simulink model "k1vispr2"  (Simulink 8.8)
settings: Solver=ode45  StartTime=0.0  StopTime=10.0  RelTol=1e-3  EnableMultiTasking=on
libraries: cdsEpicsBinIn x38, cdsEpicsOut x14, cdsBit2Word x14, cdsIPCx x12, cdsCDI64 x7, cdsCDO64 x7, cdsWord2Bit x6, dac x2, cdsAdcx0 x1, cdsCDO32 x1, TYPEBP_MASTER x1, BO_TYPEBP_MASTER x1
(part 2 of 3)

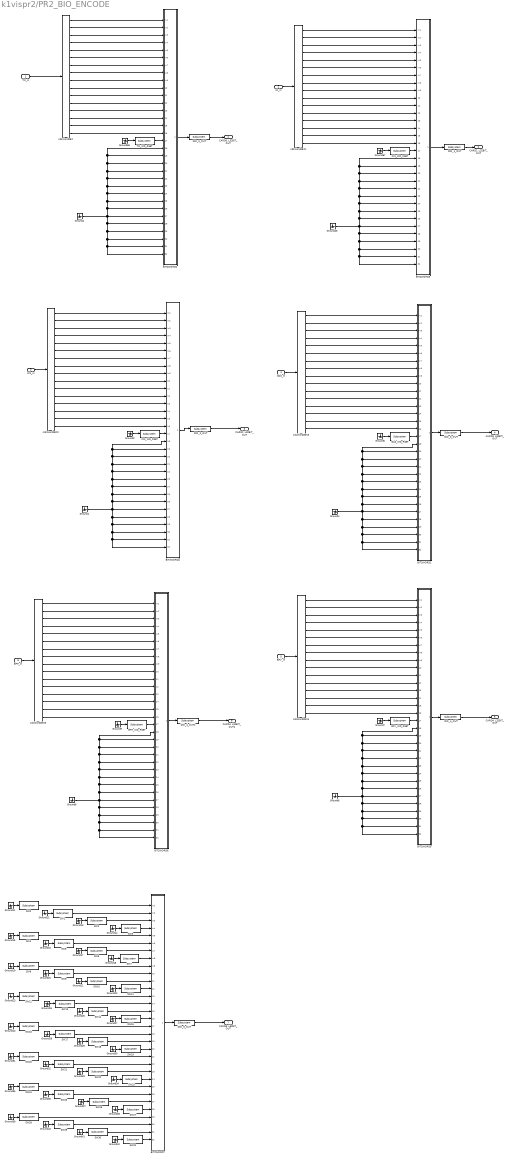
== system k1vispr2/PR2_BIO_ENCODE ==
  TM_In : Inport
  IM_In : Inport  Port=2
  IM1_In : Inport  Port=3
  GAS_In : Inport  Port=4
  BFV_In : Inport  Port=5
  BFH_In : Inport  Port=6
  BFH_WD_RSET : cdsEpicsBinIn/Subsystem  Tag=cdsEpicsBinIn  Description=|
      | Purpose:                                                                            
      | Create an EPICS binary (0 or 1) input channel to the FE realtime controls.          
      |                                                                                     
      | Operation:                                                                          
      | Outputs value from an EPICS ai record. Value is binary input (bi Epics record type).
      |                                                                                     
      | Usage:                                                                              
      | Name the part with the desired EPICS channel name.
      settings: AttributesFormatString=%<Tag>
  BFV_WD_RSET : cdsEpicsBinIn/Subsystem  Tag=cdsEpicsBinIn  Description=|
      | Purpose:                                                                            
      | Create an EPICS binary (0 or 1) input channel to the FE realtime controls.          
      |                                                                                     
      | Operation:                                                                          
      | Outputs value from an EPICS ai record. Value is binary input (bi Epics record type).
      |                                                                                     
      | Usage:                                                                              
      | Name the part with the desired EPICS channel name.
      settings: AttributesFormatString=%<Tag>
  BIT2WORD1 : Subsystem
  BIT2WORD2 : Subsystem
  BIT2WORD3 : Subsystem
  BIT2WORD4 : Subsystem
  BIT2WORD5 : Subsystem
  BIT2WORD6 : Subsystem
  BIT2WORD7 : Subsystem
  DIO_0_OUT : cdsEpicsOut/Subsystem  Tag=cdsEpicsOutput  Description=|
      | Purpose:                                          
      | Output a FE signal to an EPICS channel.           
      |                                                   
      | Operation:                                        
      | Takes input value and passes it to EPICS record.  
      |                                                   
      | Usage:                                            
      | Name the part with the desired EPICS rrecord name.
      settings: AttributesFormatString=%<Tag>
  DIO_1_OUT : cdsEpicsOut/Subsystem  Tag=cdsEpicsOutput  Description=|
      | Purpose:                                          
      | Output a FE signal to an EPICS channel.           
      |                                                   
      | Operation:                                        
      | Takes input value and passes it to EPICS record.  
      |                                                   
      | Usage:                                            
      | Name the part with the desired EPICS rrecord name.
      settings: AttributesFormatString=%<Tag>
  DIO_2_OUT : cdsEpicsOut/Subsystem  Tag=cdsEpicsOutput  Description=|
      | Purpose:                                          
      | Output a FE signal to an EPICS channel.           
      |                                                   
      | Operation:                                        
      | Takes input value and passes it to EPICS record.  
      |                                                   
      | Usage:                                            
      | Name the part with the desired EPICS rrecord name.
      settings: AttributesFormatString=%<Tag>
  DIO_3_OUT : cdsEpicsOut/Subsystem  Tag=cdsEpicsOutput  Description=|
      | Purpose:                                          
      | Output a FE signal to an EPICS channel.           
      |                                                   
      | Operation:                                        
      | Takes input value and passes it to EPICS record.  
      |                                                   
      | Usage:                                            
      | Name the part with the desired EPICS rrecord name.
      settings: AttributesFormatString=%<Tag>
  DIO_4_OUT : cdsEpicsOut/Subsystem  Tag=cdsEpicsOutput  Description=|
      | Purpose:                                          
      | Output a FE signal to an EPICS channel.           
      |                                                   
      | Operation:                                        
      | Takes input value and passes it to EPICS record.  
      |                                                   
      | Usage:                                            
      | Name the part with the desired EPICS rrecord name.
      settings: AttributesFormatString=%<Tag>
  DIO_4_OUT1 : cdsEpicsOut/Subsystem  Tag=cdsEpicsOutput  Description=|
      | Purpose:                                          
      | Output a FE signal to an EPICS channel.           
      |                                                   
      | Operation:                                        
      | Takes input value and passes it to EPICS record.  
      |                                                   
      | Usage:                                            
      | Name the part with the desired EPICS rrecord name.
      settings: AttributesFormatString=%<Tag>
  DIO_6_OUT : cdsEpicsOut/Subsystem  Tag=cdsEpicsOutput  Description=|
      | Purpose:                                          
      | Output a FE signal to an EPICS channel.           
      |                                                   
      | Operation:                                        
      | Takes input value and passes it to EPICS record.  
      |                                                   
      | Usage:                                            
      | Name the part with the desired EPICS rrecord name.
      settings: AttributesFormatString=%<Tag>
  GAS_WD_RSET : cdsEpicsBinIn/Subsystem  Tag=cdsEpicsBinIn  Description=|
      | Purpose:                                                                            
      | Create an EPICS binary (0 or 1) input channel to the FE realtime controls.          
      |                                                                                     
      | Operation:                                                                          
      | Outputs value from an EPICS ai record. Value is binary input (bi Epics record type).
      |                                                                                     
      | Usage:                                                                              
      | Name the part with the desired EPICS channel name.
      settings: AttributesFormatString=%<Tag>
  Ground{1..42,66..67} (44 alike) : Ground
  IM1_WD_RSET : cdsEpicsBinIn/Subsystem  Tag=cdsEpicsBinIn  Description=|
      | Purpose:                                                                            
      | Create an EPICS binary (0 or 1) input channel to the FE realtime controls.          
      |                                                                                     
      | Operation:                                                                          
      | Outputs value from an EPICS ai record. Value is binary input (bi Epics record type).
      |                                                                                     
      | Usage:                                                                              
      | Name the part with the desired EPICS channel name.
      settings: AttributesFormatString=%<Tag>
  IM2_WD_RSET : cdsEpicsBinIn/Subsystem  Tag=cdsEpicsBinIn  Description=|
      | Purpose:                                                                            
      | Create an EPICS binary (0 or 1) input channel to the FE realtime controls.          
      |                                                                                     
      | Operation:                                                                          
      | Outputs value from an EPICS ai record. Value is binary input (bi Epics record type).
      |                                                                                     
      | Usage:                                                                              
      | Name the part with the desired EPICS channel name.
      settings: AttributesFormatString=%<Tag>
  SW0 : cdsEpicsBinIn/Subsystem  Tag=cdsEpicsBinIn  Description=|
      | Purpose:                                                                            
      | Create an EPICS binary (0 or 1) input channel to the FE realtime controls.          
      |                                                                                     
      | Operation:                                                                          
      | Outputs value from an EPICS ai record. Value is binary input (bi Epics record type).
      |                                                                                     
      | Usage:                                                                              
      | Name the part with the desired EPICS channel name.
      settings: AttributesFormatString=%<Tag>
  SW1 : cdsEpicsBinIn/Subsystem  Tag=cdsEpicsBinIn  Description=|
      | Purpose:                                                                            
      | Create an EPICS binary (0 or 1) input channel to the FE realtime controls.          
      |                                                                                     
      | Operation:                                                                          
      | Outputs value from an EPICS ai record. Value is binary input (bi Epics record type).
      |                                                                                     
      | Usage:                                                                              
      | Name the part with the desired EPICS channel name.
      settings: AttributesFormatString=%<Tag>
  SW10 : cdsEpicsBinIn/Subsystem  Tag=cdsEpicsBinIn  Description=|
      | Purpose:                                                                            
      | Create an EPICS binary (0 or 1) input channel to the FE realtime controls.          
      |                                                                                     
      | Operation:                                                                          
      | Outputs value from an EPICS ai record. Value is binary input (bi Epics record type).
      |                                                                                     
      | Usage:                                                                              
      | Name the part with the desired EPICS channel name.
      settings: AttributesFormatString=%<Tag>
  SW11 : cdsEpicsBinIn/Subsystem  Tag=cdsEpicsBinIn  Description=|
      | Purpose:                                                                            
      | Create an EPICS binary (0 or 1) input channel to the FE realtime controls.          
      |                                                                                     
      | Operation:                                                                          
      | Outputs value from an EPICS ai record. Value is binary input (bi Epics record type).
      |                                                                                     
      | Usage:                                                                              
      | Name the part with the desired EPICS channel name.
      settings: AttributesFormatString=%<Tag>
  SW12 : cdsEpicsBinIn/Subsystem  Tag=cdsEpicsBinIn  Description=|
      | Purpose:                                                                            
      | Create an EPICS binary (0 or 1) input channel to the FE realtime controls.          
      |                                                                                     
      | Operation:                                                                          
      | Outputs value from an EPICS ai record. Value is binary input (bi Epics record type).
      |                                                                                     
      | Usage:                                                                              
      | Name the part with the desired EPICS channel name.
      settings: AttributesFormatString=%<Tag>
  SW13 : cdsEpicsBinIn/Subsystem  Tag=cdsEpicsBinIn  Description=|
      | Purpose:                                                                            
      | Create an EPICS binary (0 or 1) input channel to the FE realtime controls.          
      |                                                                                     
      | Operation:                                                                          
      | Outputs value from an EPICS ai record. Value is binary input (bi Epics record type).
      |                                                                                     
      | Usage:                                                                              
      | Name the part with the desired EPICS channel name.
      settings: AttributesFormatString=%<Tag>
  SW14 : cdsEpicsBinIn/Subsystem  Tag=cdsEpicsBinIn  Description=|
      | Purpose:                                                                            
      | Create an EPICS binary (0 or 1) input channel to the FE realtime controls.          
      |                                                                                     
      | Operation:                                                                          
      | Outputs value from an EPICS ai record. Value is binary input (bi Epics record type).
      |                                                                                     
      | Usage:                                                                              
      | Name the part with the desired EPICS channel name.
      settings: AttributesFormatString=%<Tag>
  SW15 : cdsEpicsBinIn/Subsystem  Tag=cdsEpicsBinIn  Description=|
      | Purpose:                                                                            
      | Create an EPICS binary (0 or 1) input channel to the FE realtime controls.          
      |                                                                                     
      | Operation:                                                                          
      | Outputs value from an EPICS ai record. Value is binary input (bi Epics record type).
      |                                                                                     
      | Usage:                                                                              
      | Name the part with the desired EPICS channel name.
      settings: AttributesFormatString=%<Tag>
  SW16 : cdsEpicsBinIn/Subsystem  Tag=cdsEpicsBinIn  Description=|
      | Purpose:                                                                            
      | Create an EPICS binary (0 or 1) input channel to the FE realtime controls.          
      |                                                                                     
      | Operation:                                                                          
      | Outputs value from an EPICS ai record. Value is binary input (bi Epics record type).
      |                                                                                     
      | Usage:                                                                              
      | Name the part with the desired EPICS channel name.
      settings: AttributesFormatString=%<Tag>
  SW17 : cdsEpicsBinIn/Subsystem  Tag=cdsEpicsBinIn  Description=|
      | Purpose:                                                                            
      | Create an EPICS binary (0 or 1) input channel to the FE realtime controls.          
      |                                                                                     
      | Operation:                                                                          
      | Outputs value from an EPICS ai record. Value is binary input (bi Epics record type).
      |                                                                                     
      | Usage:                                                                              
      | Name the part with the desired EPICS channel name.
      settings: AttributesFormatString=%<Tag>
  SW18 : cdsEpicsBinIn/Subsystem  Tag=cdsEpicsBinIn  Description=|
      | Purpose:                                                                            
      | Create an EPICS binary (0 or 1) input channel to the FE realtime controls.          
      |                                                                                     
      | Operation:                                                                          
      | Outputs value from an EPICS ai record. Value is binary input (bi Epics record type).
      |                                                                                     
      | Usage:                                                                              
      | Name the part with the desired EPICS channel name.
      settings: AttributesFormatString=%<Tag>
  SW19 : cdsEpicsBinIn/Subsystem  Tag=cdsEpicsBinIn  Description=|
      | Purpose:                                                                            
      | Create an EPICS binary (0 or 1) input channel to the FE realtime controls.          
      |                                                                                     
      | Operation:                                                                          
      | Outputs value from an EPICS ai record. Value is binary input (bi Epics record type).
      |                                                                                     
      | Usage:                                                                              
      | Name the part with the desired EPICS channel name.
      settings: AttributesFormatString=%<Tag>
  SW2 : cdsEpicsBinIn/Subsystem  Tag=cdsEpicsBinIn  Description=|
      | Purpose:                                                                            
      | Create an EPICS binary (0 or 1) input channel to the FE realtime controls.          
      |                                                                                     
      | Operation:                                                                          
      | Outputs value from an EPICS ai record. Value is binary input (bi Epics record type).
      |                                                                                     
      | Usage:                                                                              
      | Name the part with the desired EPICS channel name.
      settings: AttributesFormatString=%<Tag>
  SW20 : cdsEpicsBinIn/Subsystem  Tag=cdsEpicsBinIn  Description=|
      | Purpose:                                                                            
      | Create an EPICS binary (0 or 1) input channel to the FE realtime controls.          
      |                                                                                     
      | Operation:                                                                          
      | Outputs value from an EPICS ai record. Value is binary input (bi Epics record type).
      |                                                                                     
      | Usage:                                                                              
      | Name the part with the desired EPICS channel name.
      settings: AttributesFormatString=%<Tag>
  SW21 : cdsEpicsBinIn/Subsystem  Tag=cdsEpicsBinIn  Description=|
      | Purpose:                                                                            
      | Create an EPICS binary (0 or 1) input channel to the FE realtime controls.          
      |                                                                                     
      | Operation:                                                                          
      | Outputs value from an EPICS ai record. Value is binary input (bi Epics record type).
      |                                                                                     
      | Usage:                                                                              
      | Name the part with the desired EPICS channel name.
      settings: AttributesFormatString=%<Tag>
  SW22 : cdsEpicsBinIn/Subsystem  Tag=cdsEpicsBinIn  Description=|
      | Purpose:                                                                            
      | Create an EPICS binary (0 or 1) input channel to the FE realtime controls.          
      |                                                                                     
      | Operation:                                                                          
      | Outputs value from an EPICS ai record. Value is binary input (bi Epics record type).
      |                                                                                     
      | Usage:                                                                              
      | Name the part with the desired EPICS channel name.
      settings: AttributesFormatString=%<Tag>
  SW23 : cdsEpicsBinIn/Subsystem  Tag=cdsEpicsBinIn  Description=|
      | Purpose:                                                                            
      | Create an EPICS binary (0 or 1) input channel to the FE realtime controls.          
      |                                                                                     
      | Operation:                                                                          
      | Outputs value from an EPICS ai record. Value is binary input (bi Epics record type).
      |                                                                                     
      | Usage:                                                                              
      | Name the part with the desired EPICS channel name.
      settings: AttributesFormatString=%<Tag>
  SW24 : cdsEpicsBinIn/Subsystem  Tag=cdsEpicsBinIn  Description=|
      | Purpose:                                                                            
      | Create an EPICS binary (0 or 1) input channel to the FE realtime controls.          
      |                                                                                     
      | Operation:                                                                          
      | Outputs value from an EPICS ai record. Value is binary input (bi Epics record type).
      |                                                                                     
      | Usage:                                                                              
      | Name the part with the desired EPICS channel name.
      settings: AttributesFormatString=%<Tag>
  SW25 : cdsEpicsBinIn/Subsystem  Tag=cdsEpicsBinIn  Description=|
      | Purpose:                                                                            
      | Create an EPICS binary (0 or 1) input channel to the FE realtime controls.          
      |                                                                                     
      | Operation:                                                                          
      | Outputs value from an EPICS ai record. Value is binary input (bi Epics record type).
      |                                                                                     
      | Usage:                                                                              
      | Name the part with the desired EPICS channel name.
      settings: AttributesFormatString=%<Tag>
  SW26 : cdsEpicsBinIn/Subsystem  Tag=cdsEpicsBinIn  Description=|
      | Purpose:                                                                            
      | Create an EPICS binary (0 or 1) input channel to the FE realtime controls.          
      |                                                                                     
      | Operation:                                                                          
      | Outputs value from an EPICS ai record. Value is binary input (bi Epics record type).
      |                                                                                     
      | Usage:                                                                              
      | Name the part with the desired EPICS channel name.
      settings: AttributesFormatString=%<Tag>
  SW27 : cdsEpicsBinIn/Subsystem  Tag=cdsEpicsBinIn  Description=|
      | Purpose:                                                                            
      | Create an EPICS binary (0 or 1) input channel to the FE realtime controls.          
      |                                                                                     
      | Operation:                                                                          
      | Outputs value from an EPICS ai record. Value is binary input (bi Epics record type).
      |                                                                                     
      | Usage:                                                                              
      | Name the part with the desired EPICS channel name.
      settings: AttributesFormatString=%<Tag>
  SW28 : cdsEpicsBinIn/Subsystem  Tag=cdsEpicsBinIn  Description=|
      | Purpose:                                                                            
      | Create an EPICS binary (0 or 1) input channel to the FE realtime controls.          
      |                                                                                     
      | Operation:                                                                          
      | Outputs value from an EPICS ai record. Value is binary input (bi Epics record type).
      |                                                                                     
      | Usage:                                                                              
      | Name the part with the desired EPICS channel name.
      settings: AttributesFormatString=%<Tag>
  SW29 : cdsEpicsBinIn/Subsystem  Tag=cdsEpicsBinIn  Description=|
      | Purpose:                                                                            
      | Create an EPICS binary (0 or 1) input channel to the FE realtime controls.          
      |                                                                                     
      | Operation:                                                                          
      | Outputs value from an EPICS ai record. Value is binary input (bi Epics record type).
      |                                                                                     
      | Usage:                                                                              
      | Name the part with the desired EPICS channel name.
      settings: AttributesFormatString=%<Tag>
  SW3 : cdsEpicsBinIn/Subsystem  Tag=cdsEpicsBinIn  Description=|
      | Purpose:                                                                            
      | Create an EPICS binary (0 or 1) input channel to the FE realtime controls.          
      |                                                                                     
      | Operation:                                                                          
      | Outputs value from an EPICS ai record. Value is binary input (bi Epics record type).
      |                                                                                     
      | Usage:                                                                              
      | Name the part with the desired EPICS channel name.
      settings: AttributesFormatString=%<Tag>
  SW30 : cdsEpicsBinIn/Subsystem  Tag=cdsEpicsBinIn  Description=|
      | Purpose:                                                                            
      | Create an EPICS binary (0 or 1) input channel to the FE realtime controls.          
      |                                                                                     
      | Operation:                                                                          
      | Outputs value from an EPICS ai record. Value is binary input (bi Epics record type).
      |                                                                                     
      | Usage:                                                                              
      | Name the part with the desired EPICS channel name.
      settings: AttributesFormatString=%<Tag>
  SW31 : cdsEpicsBinIn/Subsystem  Tag=cdsEpicsBinIn  Description=|
      | Purpose:                                                                            
      | Create an EPICS binary (0 or 1) input channel to the FE realtime controls.          
      |                                                                                     
      | Operation:                                                                          
      | Outputs value from an EPICS ai record. Value is binary input (bi Epics record type).
      |                                                                                     
      | Usage:                                                                              
      | Name the part with the desired EPICS channel name.
      settings: AttributesFormatString=%<Tag>
  SW4 : cdsEpicsBinIn/Subsystem  Tag=cdsEpicsBinIn  Description=|
      | Purpose:                                                                            
      | Create an EPICS binary (0 or 1) input channel to the FE realtime controls.          
      |                                                                                     
      | Operation:                                                                          
      | Outputs value from an EPICS ai record. Value is binary input (bi Epics record type).
      |                                                                                     
      | Usage:                                                                              
      | Name the part with the desired EPICS channel name.
      settings: AttributesFormatString=%<Tag>
  SW5 : cdsEpicsBinIn/Subsystem  Tag=cdsEpicsBinIn  Description=|
      | Purpose:                                                                            
      | Create an EPICS binary (0 or 1) input channel to the FE realtime controls.          
      |                                                                                     
      | Operation:                                                                          
      | Outputs value from an EPICS ai record. Value is binary input (bi Epics record type).
      |                                                                                     
      | Usage:                                                                              
      | Name the part with the desired EPICS channel name.
      settings: AttributesFormatString=%<Tag>
  SW6 : cdsEpicsBinIn/Subsystem  Tag=cdsEpicsBinIn  Description=|
      | Purpose:                                                                            
      | Create an EPICS binary (0 or 1) input channel to the FE realtime controls.          
      |                                                                                     
      | Operation:                                                                          
      | Outputs value from an EPICS ai record. Value is binary input (bi Epics record type).
      |                                                                                     
      | Usage:                                                                              
      | Name the part with the desired EPICS channel name.
      settings: AttributesFormatString=%<Tag>
  SW7 : cdsEpicsBinIn/Subsystem  Tag=cdsEpicsBinIn  Description=|
      | Purpose:                                                                            
      | Create an EPICS binary (0 or 1) input channel to the FE realtime controls.          
      |                                                                                     
      | Operation:                                                                          
      | Outputs value from an EPICS ai record. Value is binary input (bi Epics record type).
      |                                                                                     
      | Usage:                                                                              
      | Name the part with the desired EPICS channel name.
      settings: AttributesFormatString=%<Tag>
  SW8 : cdsEpicsBinIn/Subsystem  Tag=cdsEpicsBinIn  Description=|
      | Purpose:                                                                            
      | Create an EPICS binary (0 or 1) input channel to the FE realtime controls.          
      |                                                                                     
      | Operation:                                                                          
      | Outputs value from an EPICS ai record. Value is binary input (bi Epics record type).
      |                                                                                     
      | Usage:                                                                              
      | Name the part with the desired EPICS channel name.
      settings: AttributesFormatString=%<Tag>
  SW9 : cdsEpicsBinIn/Subsystem  Tag=cdsEpicsBinIn  Description=|
      | Purpose:                                                                            
      | Create an EPICS binary (0 or 1) input channel to the FE realtime controls.          
      |                                                                                     
      | Operation:                                                                          
      | Outputs value from an EPICS ai record. Value is binary input (bi Epics record type).
      |                                                                                     
      | Usage:                                                                              
      | Name the part with the desired EPICS channel name.
      settings: AttributesFormatString=%<Tag>
  TM_WD_RSET : cdsEpicsBinIn/Subsystem  Tag=cdsEpicsBinIn  Description=|
      | Purpose:                                                                            
      | Create an EPICS binary (0 or 1) input channel to the FE realtime controls.          
      |                                                                                     
      | Operation:                                                                          
      | Outputs value from an EPICS ai record. Value is binary input (bi Epics record type).
      |                                                                                     
      | Usage:                                                                              
      | Name the part with the desired EPICS channel name.
      settings: AttributesFormatString=%<Tag>
  cdsWord2Bit{,1..5} (6 alike) : cdsWord2Bit/cdsWord2Bit  Tag=cdsWord2Bit  Description=Generate 16 0/1 outputs from single 16-bit integer input
      settings: AttributesFormatString=cdsWord2Bit
  CARD0_L32BIT_OUT : Outport
  CARD1_L32BIT_OUT : Outport  Port=2
  CARD2_L32BIT_OUT : Outport  Port=3
  CARD3_L32BIT_OUT : Outport  Port=4
  CARD4_L32BIT_OUT : Outport  Port=5
  CARD4_L32BIT_OUT1 : Outport  Port=6
  CARD6_L32BIT_OUT : Outport  Port=7
  wires:
  Ground2/1 -> BIT2WORD2/20(In20), BIT2WORD2/18(In18), BIT2WORD2/19(In19), BIT2WORD2/21(In21), BIT2WORD2/22(In22), BIT2WORD2/23(In23), BIT2WORD2/24(In24), BIT2WORD2/25(In25), BIT2WORD2/26(In26), BIT2WORD2/28(In28), BIT2WORD2/31(In31), BIT2WORD2/32(In32), BIT2WORD2/30(In30), BIT2WORD2/29(In29), BIT2WORD2/27(In27)
  TM_In/1 -> cdsWord2Bit/1
  cdsWord2Bit/4 -> BIT2WORD2/4(In4)
  cdsWord2Bit/5 -> BIT2WORD2/5(In5)
  cdsWord2Bit/3 -> BIT2WORD2/3(In3)
  cdsWord2Bit/2 -> BIT2WORD2/2(In2)
  cdsWord2Bit/6 -> BIT2WORD2/6(In6)
  cdsWord2Bit/1 -> BIT2WORD2/1(In1)
  cdsWord2Bit/7 -> BIT2WORD2/7(In7)
  cdsWord2Bit/8 -> BIT2WORD2/8(In8)
  cdsWord2Bit/9 -> BIT2WORD2/9(In9)
  cdsWord2Bit/10 -> BIT2WORD2/10(In10)
  cdsWord2Bit/11 -> BIT2WORD2/11(In11)
  Ground26/1 -> BIT2WORD3/20(In20), BIT2WORD3/18(In18), BIT2WORD3/19(In19), BIT2WORD3/21(In21), BIT2WORD3/22(In22), BIT2WORD3/23(In23), BIT2WORD3/24(In24), BIT2WORD3/25(In25), BIT2WORD3/26(In26), BIT2WORD3/28(In28), BIT2WORD3/31(In31), BIT2WORD3/32(In32), BIT2WORD3/30(In30), BIT2WORD3/29(In29), BIT2WORD3/27(In27)
  IM_In/1 -> cdsWord2Bit1/1
  cdsWord2Bit1/4 -> BIT2WORD3/4(In4)
  cdsWord2Bit1/5 -> BIT2WORD3/5(In5)
  cdsWord2Bit1/3 -> BIT2WORD3/3(In3)
  cdsWord2Bit1/2 -> BIT2WORD3/2(In2)
  cdsWord2Bit1/6 -> BIT2WORD3/6(In6)
  cdsWord2Bit1/1 -> BIT2WORD3/1(In1)
  cdsWord2Bit1/7 -> BIT2WORD3/7(In7)
  cdsWord2Bit1/8 -> BIT2WORD3/8(In8)
  cdsWord2Bit1/9 -> BIT2WORD3/9(In9)
  cdsWord2Bit1/10 -> BIT2WORD3/10(In10)
  cdsWord2Bit1/11 -> BIT2WORD3/11(In11)
  Ground66/1 -> TM_WD_RSET/1
  Ground67/1 -> IM1_WD_RSET/1
  TM_WD_RSET/1 -> BIT2WORD2/17(In17)
  IM1_WD_RSET/1 -> BIT2WORD3/17(In17)
  DIO_0_OUT/1 -> CARD0_L32BIT_OUT/1
  DIO_2_OUT/1 -> CARD2_L32BIT_OUT/1
  BIT2WORD2/1(Out1) -> DIO_0_OUT/1
  BIT2WORD3/1(Out1) -> DIO_1_OUT/1
  DIO_1_OUT/1 -> CARD1_L32BIT_OUT/1
  BIT2WORD4/1(Out1) -> DIO_2_OUT/1
  BIT2WORD1/1(Out1) -> DIO_3_OUT/1
  DIO_3_OUT/1 -> CARD3_L32BIT_OUT/1
  Ground1/1 -> BIT2WORD4/27(In27), BIT2WORD4/26(In26), BIT2WORD4/25(In25), BIT2WORD4/24(In24), BIT2WORD4/23(In23), BIT2WORD4/22(In22), BIT2WORD4/21(In21), BIT2WORD4/20(In20), BIT2WORD4/19(In19), BIT2WORD4/18(In18), BIT2WORD4/28(In28), BIT2WORD4/29(In29), BIT2WORD4/30(In30), BIT2WORD4/32(In32), BIT2WORD4/31(In31)
  IM1_In/1 -> cdsWord2Bit2/1
  cdsWord2Bit2/4 -> BIT2WORD4/4(In4)
  cdsWord2Bit2/5 -> BIT2WORD4/5(In5)
  cdsWord2Bit2/3 -> BIT2WORD4/3(In3)
  cdsWord2Bit2/2 -> BIT2WORD4/2(In2)
  cdsWord2Bit2/6 -> BIT2WORD4/6(In6)
  cdsWord2Bit2/1 -> BIT2WORD4/1(In1)
  cdsWord2Bit2/7 -> BIT2WORD4/7(In7)
  cdsWord2Bit2/8 -> BIT2WORD4/8(In8)
  cdsWord2Bit2/9 -> BIT2WORD4/9(In9)
  cdsWord2Bit2/10 -> BIT2WORD4/10(In10)
  cdsWord2Bit2/11 -> BIT2WORD4/11(In11)
  Ground3/1 -> IM2_WD_RSET/1
  IM2_WD_RSET/1 -> BIT2WORD4/17(In17)
  Ground4/1 -> BIT2WORD1/27(In27), BIT2WORD1/26(In26), BIT2WORD1/25(In25), BIT2WORD1/24(In24), BIT2WORD1/23(In23), BIT2WORD1/22(In22), BIT2WORD1/21(In21), BIT2WORD1/20(In20), BIT2WORD1/19(In19), BIT2WORD1/18(In18), BIT2WORD1/28(In28), BIT2WORD1/29(In29), BIT2WORD1/30(In30), BIT2WORD1/32(In32), BIT2WORD1/31(In31)
  GAS_In/1 -> cdsWord2Bit3/1
  cdsWord2Bit3/4 -> BIT2WORD1/4(In4)
  cdsWord2Bit3/5 -> BIT2WORD1/5(In5)
  cdsWord2Bit3/3 -> BIT2WORD1/3(In3)
  cdsWord2Bit3/2 -> BIT2WORD1/2(In2)
  cdsWord2Bit3/6 -> BIT2WORD1/6(In6)
  cdsWord2Bit3/1 -> BIT2WORD1/1(In1)
  cdsWord2Bit3/7 -> BIT2WORD1/7(In7)
  cdsWord2Bit3/8 -> BIT2WORD1/8(In8)
  cdsWord2Bit3/9 -> BIT2WORD1/9(In9)
  cdsWord2Bit3/10 -> BIT2WORD1/10(In10)
  cdsWord2Bit3/11 -> BIT2WORD1/11(In11)
  Ground5/1 -> GAS_WD_RSET/1
  GAS_WD_RSET/1 -> BIT2WORD1/17(In17)
  cdsWord2Bit/12 -> BIT2WORD2/12(In12)
  cdsWord2Bit/13 -> BIT2WORD2/13(In13)
  cdsWord2Bit/14 -> BIT2WORD2/14(In14)
  cdsWord2Bit/15 -> BIT2WORD2/15(In15)
  cdsWord2Bit/16 -> BIT2WORD2/16(In16)
  cdsWord2Bit1/12 -> BIT2WORD3/12(In12)
  cdsWord2Bit1/16 -> BIT2WORD3/16(In16)
  cdsWord2Bit1/14 -> BIT2WORD3/14(In14)
  cdsWord2Bit1/15 -> BIT2WORD3/15(In15)
  cdsWord2Bit1/13 -> BIT2WORD3/13(In13)
  cdsWord2Bit3/13 -> BIT2WORD1/13(In13)
  cdsWord2Bit3/14 -> BIT2WORD1/14(In14)
  cdsWord2Bit3/15 -> BIT2WORD1/15(In15)
  cdsWord2Bit3/16 -> BIT2WORD1/16(In16)
  cdsWord2Bit3/12 -> BIT2WORD1/12(In12)
  cdsWord2Bit2/13 -> BIT2WORD4/13(In13)
  cdsWord2Bit2/15 -> BIT2WORD4/15(In15)
  cdsWord2Bit2/14 -> BIT2WORD4/14(In14)
  cdsWord2Bit2/12 -> BIT2WORD4/12(In12)
  cdsWord2Bit2/16 -> BIT2WORD4/16(In16)
  BIT2WORD5/1(Out1) -> DIO_4_OUT/1
  DIO_4_OUT/1 -> CARD4_L32BIT_OUT/1
  Ground6/1 -> BIT2WORD5/27(In27), BIT2WORD5/26(In26), BIT2WORD5/25(In25), BIT2WORD5/24(In24), BIT2WORD5/23(In23), BIT2WORD5/22(In22), BIT2WORD5/21(In21), BIT2WORD5/20(In20), BIT2WORD5/19(In19), BIT2WORD5/18(In18), BIT2WORD5/28(In28), BIT2WORD5/29(In29), BIT2WORD5/30(In30), BIT2WORD5/32(In32), BIT2WORD5/31(In31)
  BFV_In/1 -> cdsWord2Bit4/1
  cdsWord2Bit4/4 -> BIT2WORD5/4(In4)
  cdsWord2Bit4/5 -> BIT2WORD5/5(In5)
  cdsWord2Bit4/3 -> BIT2WORD5/3(In3)
  cdsWord2Bit4/2 -> BIT2WORD5/2(In2)
  cdsWord2Bit4/6 -> BIT2WORD5/6(In6)
  cdsWord2Bit4/1 -> BIT2WORD5/1(In1)
  cdsWord2Bit4/7 -> BIT2WORD5/7(In7)
  cdsWord2Bit4/8 -> BIT2WORD5/8(In8)
  cdsWord2Bit4/9 -> BIT2WORD5/9(In9)
  cdsWord2Bit4/10 -> BIT2WORD5/10(In10)
  cdsWord2Bit4/11 -> BIT2WORD5/11(In11)
  Ground7/1 -> BFV_WD_RSET/1
  BFV_WD_RSET/1 -> BIT2WORD5/17(In17)
  cdsWord2Bit4/13 -> BIT2WORD5/13(In13)
  cdsWord2Bit4/14 -> BIT2WORD5/14(In14)
  cdsWord2Bit4/15 -> BIT2WORD5/15(In15)
  cdsWord2Bit4/16 -> BIT2WORD5/16(In16)
  cdsWord2Bit4/12 -> BIT2WORD5/12(In12)
  BIT2WORD6/1(Out1) -> DIO_4_OUT1/1
  DIO_4_OUT1/1 -> CARD4_L32BIT_OUT1/1
  Ground8/1 -> BIT2WORD6/27(In27), BIT2WORD6/26(In26), BIT2WORD6/25(In25), BIT2WORD6/24(In24), BIT2WORD6/23(In23), BIT2WORD6/22(In22), BIT2WORD6/21(In21), BIT2WORD6/20(In20), BIT2WORD6/19(In19), BIT2WORD6/18(In18), BIT2WORD6/28(In28), BIT2WORD6/29(In29), BIT2WORD6/30(In30), BIT2WORD6/32(In32), BIT2WORD6/31(In31)
  BFH_In/1 -> cdsWord2Bit5/1
  cdsWord2Bit5/4 -> BIT2WORD6/4(In4)
  cdsWord2Bit5/5 -> BIT2WORD6/5(In5)
  cdsWord2Bit5/3 -> BIT2WORD6/3(In3)
  cdsWord2Bit5/2 -> BIT2WORD6/2(In2)
  cdsWord2Bit5/6 -> BIT2WORD6/6(In6)
  cdsWord2Bit5/1 -> BIT2WORD6/1(In1)
  cdsWord2Bit5/7 -> BIT2WORD6/7(In7)
  cdsWord2Bit5/8 -> BIT2WORD6/8(In8)
  cdsWord2Bit5/9 -> BIT2WORD6/9(In9)
  cdsWord2Bit5/10 -> BIT2WORD6/10(In10)
  cdsWord2Bit5/11 -> BIT2WORD6/11(In11)
  Ground9/1 -> BFH_WD_RSET/1
  BFH_WD_RSET/1 -> BIT2WORD6/17(In17)
  cdsWord2Bit5/13 -> BIT2WORD6/13(In13)
  cdsWord2Bit5/14 -> BIT2WORD6/14(In14)
  cdsWord2Bit5/15 -> BIT2WORD6/15(In15)
  cdsWord2Bit5/16 -> BIT2WORD6/16(In16)
  cdsWord2Bit5/12 -> BIT2WORD6/12(In12)
  BIT2WORD7/1(Out1) -> DIO_6_OUT/1
  DIO_6_OUT/1 -> CARD6_L32BIT_OUT/1
  SW26/1 -> BIT2WORD7/27(In27)
  SW25/1 -> BIT2WORD7/26(In26)
  SW24/1 -> BIT2WORD7/25(In25)
  SW23/1 -> BIT2WORD7/24(In24)
  SW22/1 -> BIT2WORD7/23(In23)
  SW21/1 -> BIT2WORD7/22(In22)
  SW20/1 -> BIT2WORD7/21(In21)
  SW19/1 -> BIT2WORD7/20(In20)
  SW18/1 -> BIT2WORD7/19(In19)
  SW17/1 -> BIT2WORD7/18(In18)
  SW27/1 -> BIT2WORD7/28(In28)
  SW28/1 -> BIT2WORD7/29(In29)
  SW29/1 -> BIT2WORD7/30(In30)
  SW30/1 -> BIT2WORD7/31(In31)
  SW3/1 -> BIT2WORD7/4(In4)
  SW4/1 -> BIT2WORD7/5(In5)
  SW2/1 -> BIT2WORD7/3(In3)
  SW1/1 -> BIT2WORD7/2(In2)
  SW5/1 -> BIT2WORD7/6(In6)
  SW0/1 -> BIT2WORD7/1(In1)
  SW6/1 -> BIT2WORD7/7(In7)
  SW7/1 -> BIT2WORD7/8(In8)
  SW8/1 -> BIT2WORD7/9(In9)
  SW9/1 -> BIT2WORD7/10(In10)
  SW10/1 -> BIT2WORD7/11(In11)
  Ground10/1 -> SW16/1
  SW16/1 -> BIT2WORD7/17(In17)
  SW12/1 -> BIT2WORD7/13(In13)
  SW13/1 -> BIT2WORD7/14(In14)
  SW14/1 -> BIT2WORD7/15(In15)
  SW15/1 -> BIT2WORD7/16(In16)
  SW11/1 -> BIT2WORD7/12(In12)
  Ground11/1 -> SW0/1
  Ground12/1 -> SW1/1
  Ground13/1 -> SW2/1
  Ground14/1 -> SW3/1
  Ground15/1 -> SW4/1
  Ground16/1 -> SW5/1
  Ground17/1 -> SW6/1
  Ground18/1 -> SW7/1
  Ground19/1 -> SW8/1
  Ground20/1 -> SW9/1
  Ground21/1 -> SW10/1
  Ground22/1 -> SW11/1
  Ground23/1 -> SW12/1
  Ground24/1 -> SW13/1
  Ground25/1 -> SW14/1
  Ground27/1 -> SW15/1
  Ground28/1 -> SW17/1
  Ground29/1 -> SW18/1
  Ground30/1 -> SW19/1
  Ground31/1 -> SW20/1
  Ground32/1 -> SW21/1
  Ground33/1 -> SW22/1
  Ground34/1 -> SW23/1
  Ground35/1 -> SW24/1
  Ground36/1 -> SW25/1
  Ground37/1 -> SW26/1
  Ground38/1 -> SW27/1
  Ground39/1 -> SW28/1
  Ground40/1 -> SW29/1
  Ground41/1 -> SW30/1
  Ground42/1 -> SW31/1
  SW31/1 -> BIT2WORD7/32(In32)

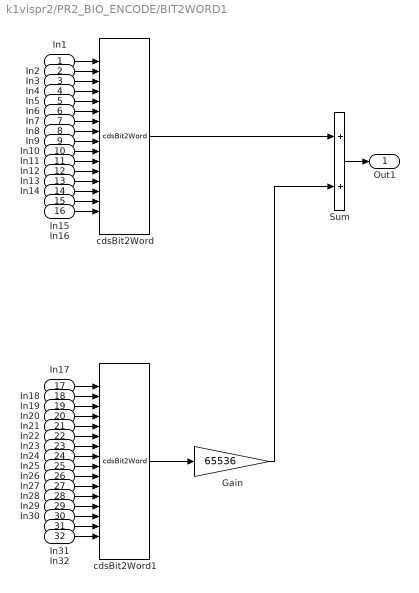
== system k1vispr2/PR2_BIO_ENCODE/BIT2WORD1 ==
  In1 : Inport
  In2 : Inport  Port=2
  In3 : Inport  Port=3
  In4 : Inport  Port=4
  In5 : Inport  Port=5
  In6 : Inport  Port=6
  In7 : Inport  Port=7
  In8 : Inport  Port=8
  In9 : Inport  Port=9
  In10 : Inport  Port=10
  In11 : Inport  Port=11
  In12 : Inport  Port=12
  In13 : Inport  Port=13
  In14 : Inport  Port=14
  In15 : Inport  Port=15
  In16 : Inport  Port=16
  In17 : Inport  Port=17
  In18 : Inport  Port=18
  In19 : Inport  Port=19
  In20 : Inport  Port=20
  In21 : Inport  Port=21
  In22 : Inport  Port=22
  In23 : Inport  Port=23
  In24 : Inport  Port=24
  In25 : Inport  Port=25
  In26 : Inport  Port=26
  In27 : Inport  Port=27
  In28 : Inport  Port=28
  In29 : Inport  Port=29
  In30 : Inport  Port=30
  In31 : Inport  Port=31
  In32 : Inport  Port=32
  Gain : Gain  Gain=65536
  Sum : Sum
  cdsBit2Word : cdsBit2Word/cdsBit2Word  Tag=cdsBit2Word  Description=Forms single 16 bit integer from 16 0/1 inputs.
      settings: AttributesFormatString=%<Tag>
  cdsBit2Word1 : cdsBit2Word/cdsBit2Word  Tag=cdsBit2Word  Description=Forms single 16 bit integer from 16 0/1 inputs.
      settings: AttributesFormatString=%<Tag>
  Out1 : Outport
  wires:
  Gain/1 -> Sum/2
  cdsBit2Word1/1 -> Gain/1
  cdsBit2Word/1 -> Sum/1
  In1/1 -> cdsBit2Word/1
  In2/1 -> cdsBit2Word/2
  In3/1 -> cdsBit2Word/3
  In4/1 -> cdsBit2Word/4
  In5/1 -> cdsBit2Word/5
  In6/1 -> cdsBit2Word/6
  In7/1 -> cdsBit2Word/7
  In8/1 -> cdsBit2Word/8
  In9/1 -> cdsBit2Word/9
  In10/1 -> cdsBit2Word/10
  Sum/1 -> Out1/1
  In11/1 -> cdsBit2Word/11
  In12/1 -> cdsBit2Word/12
  In13/1 -> cdsBit2Word/13
  In14/1 -> cdsBit2Word/14
  In15/1 -> cdsBit2Word/15
  In16/1 -> cdsBit2Word/16
  In17/1 -> cdsBit2Word1/1
  In18/1 -> cdsBit2Word1/2
  In19/1 -> cdsBit2Word1/3
  In20/1 -> cdsBit2Word1/4
  In21/1 -> cdsBit2Word1/5
  In22/1 -> cdsBit2Word1/6
  In23/1 -> cdsBit2Word1/7
  In24/1 -> cdsBit2Word1/8
  In25/1 -> cdsBit2Word1/9
  In26/1 -> cdsBit2Word1/10
  In27/1 -> cdsBit2Word1/11
  In28/1 -> cdsBit2Word1/12
  In29/1 -> cdsBit2Word1/13
  In30/1 -> cdsBit2Word1/14
  In31/1 -> cdsBit2Word1/15
  In32/1 -> cdsBit2Word1/16

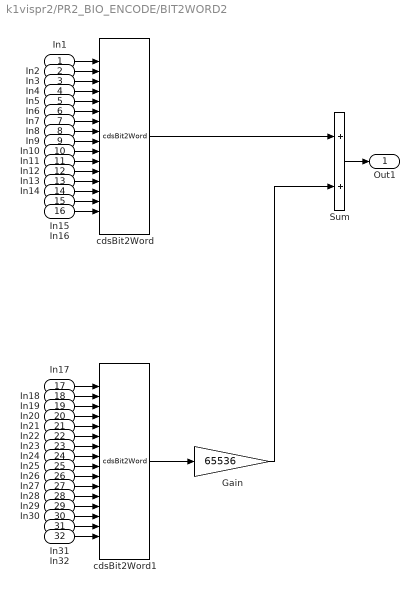
== system k1vispr2/PR2_BIO_ENCODE/BIT2WORD2 ==
  In1 : Inport
  In2 : Inport  Port=2
  In3 : Inport  Port=3
  In4 : Inport  Port=4
  In5 : Inport  Port=5
  In6 : Inport  Port=6
  In7 : Inport  Port=7
  In8 : Inport  Port=8
  In9 : Inport  Port=9
  In10 : Inport  Port=10
  In11 : Inport  Port=11
  In12 : Inport  Port=12
  In13 : Inport  Port=13
  In14 : Inport  Port=14
  In15 : Inport  Port=15
  In16 : Inport  Port=16
  In17 : Inport  Port=17
  In18 : Inport  Port=18
  In19 : Inport  Port=19
  In20 : Inport  Port=20
  In21 : Inport  Port=21
  In22 : Inport  Port=22
  In23 : Inport  Port=23
  In24 : Inport  Port=24
  In25 : Inport  Port=25
  In26 : Inport  Port=26
  In27 : Inport  Port=27
  In28 : Inport  Port=28
  In29 : Inport  Port=29
  In30 : Inport  Port=30
  In31 : Inport  Port=31
  In32 : Inport  Port=32
  Gain : Gain  Gain=65536
  Sum : Sum
  cdsBit2Word : cdsBit2Word/cdsBit2Word  Tag=cdsBit2Word  Description=Forms single 16 bit integer from 16 0/1 inputs.
      settings: AttributesFormatString=%<Tag>
  cdsBit2Word1 : cdsBit2Word/cdsBit2Word  Tag=cdsBit2Word  Description=Forms single 16 bit integer from 16 0/1 inputs.
      settings: AttributesFormatString=%<Tag>
  Out1 : Outport
  wires:
  Gain/1 -> Sum/2
  cdsBit2Word1/1 -> Gain/1
  cdsBit2Word/1 -> Sum/1
  In1/1 -> cdsBit2Word/1
  In2/1 -> cdsBit2Word/2
  In3/1 -> cdsBit2Word/3
  In4/1 -> cdsBit2Word/4
  In5/1 -> cdsBit2Word/5
  In6/1 -> cdsBit2Word/6
  In7/1 -> cdsBit2Word/7
  In8/1 -> cdsBit2Word/8
  In9/1 -> cdsBit2Word/9
  In10/1 -> cdsBit2Word/10
  Sum/1 -> Out1/1
  In11/1 -> cdsBit2Word/11
  In12/1 -> cdsBit2Word/12
  In13/1 -> cdsBit2Word/13
  In14/1 -> cdsBit2Word/14
  In15/1 -> cdsBit2Word/15
  In16/1 -> cdsBit2Word/16
  In17/1 -> cdsBit2Word1/1
  In18/1 -> cdsBit2Word1/2
  In19/1 -> cdsBit2Word1/3
  In20/1 -> cdsBit2Word1/4
  In21/1 -> cdsBit2Word1/5
  In22/1 -> cdsBit2Word1/6
  In23/1 -> cdsBit2Word1/7
  In24/1 -> cdsBit2Word1/8
  In25/1 -> cdsBit2Word1/9
  In26/1 -> cdsBit2Word1/10
  In27/1 -> cdsBit2Word1/11
  In28/1 -> cdsBit2Word1/12
  In29/1 -> cdsBit2Word1/13
  In30/1 -> cdsBit2Word1/14
  In31/1 -> cdsBit2Word1/15
  In32/1 -> cdsBit2Word1/16
